simulink model "Micro_Grid_BatteryCharging"  (R2024b)
settings: Solver=VariableStepAuto  StartTime=0.0  StopTime=60*3  RelTol=1e-3
undefined symbols (not defined in the file or in its folder): Acid, Lead
libraries: spsSeriesRLCBranchLib x15, spsVoltageMeasurementLib x9, spsThreePhaseSourceLib x3, spsUniversalBridgeLib x3, spsThreePhaseSeriesRLCBranchLib x2, spsCurrentMeasurementLib x2, spsPWMGenerator2LevelLib x2, spsBreakerLib x2, spsThreePhaseVIMeasurementLib x1, spsBatteryLib x1, slpidlib x1, spsSawtoothGeneratorLib x1
settings Model: SimulationMode=accelerator  Creator=haima  LastModifiedBy=haima

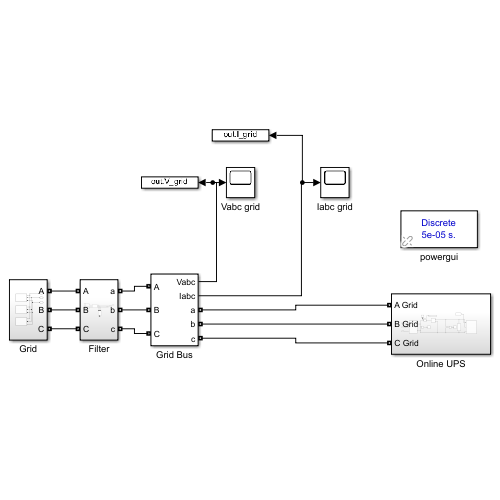
[thumbnail: Simulink's stored preview of the top-level diagram]
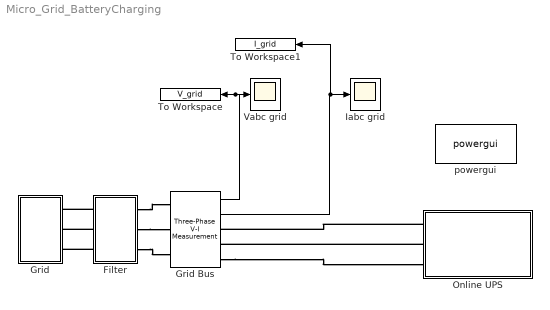
== system Micro_Grid_BatteryCharging ==
  Filter : Subsystem
  Grid : Subsystem
  Grid Bus : spsThreePhaseVIMeasurementLib/Three-Phase V-I Measurement  VoltageMeasurement=phase-to-ground  SetLabelV=off  LabelV=Vabc  Vpu=off  VpuLL=off  CurrentMeasurement=yes  SetLabelI=off  LabelI=Iabc  Ipu=off  Pbase=100e6  Vbase=500e3  OutputType=Complex  PhasorSimulation=off  PSBequivalent=0
  Iabc grid : Scope
  Online UPS : Subsystem
  To Workspace : ToWorkspace  VariableName=V_grid  SaveFormat=Timeseries  SampleTime=-1
  To Workspace1 : ToWorkspace  VariableName=I_grid  SaveFormat=Timeseries  SampleTime=-1
  Vabc grid : Scope
  powergui : spspowerguiLib/powergui  Priority=1  SimulationMode=Discrete  SampleTime=50e-6  frequency=60  Iterations=50  frequencyindice=50  Pbase=100e6  ErrMax=1e-4  UnitsV=kV  UnitsW=MW  buscounter=0  FunctionMessages=off  echomessages=off  EnableUseOfTLC=off  CurrentSourceSwitches=off  DisableSnubberDevices=off  DisableRonSwitches=off  DisableVfSwitches=off  DisplayEquations=off  AutomaticDiscreteSolvers=off  SolverType=Tustin/Backward Euler (TBE)  Interpol=off  ExternalGateDelay=off  methode=off  Ts=100  x0status=blocks  SPID=on  SwTol=0  HookPort=off  NonlinearTolerance=1e-4  nMaxIteration=100  ContinueOnMaxIteration=off  RestoreLinks=warning  ResistiveCurrentMeasurement=off  Frange=[0:2:500]  Ylog=off  Xlog=on  ShowGrid=off  save=off  variable=ZData  structure=0  ZoomFFT=off  StartTime=0.0  cycles=1  DisplayStyle=1  fundamental=60  FreqAxis=off  MaxFrequency=1000  frequencyindicesteady=1  RmsSteady=1  display=off
  wires:
  Grid Bus/2 -> To Workspace1/1, Iabc grid/1
  Grid Bus/1 -> Vabc grid/1, To Workspace/1
  connections:
  Online UPS/LConn1 -- Grid Bus/RConn1
  Grid Bus/RConn3 -- Online UPS/LConn3
  Filter/RConn1 -- Grid Bus/LConn1
  Filter/LConn2 -- Grid/RConn2
  Filter/RConn3 -- Grid Bus/LConn3
  Online UPS/LConn2 -- Grid Bus/RConn2
  Filter/LConn1 -- Grid/RConn1
  Filter/RConn2 -- Grid Bus/LConn2
  Filter/LConn3 -- Grid/RConn3

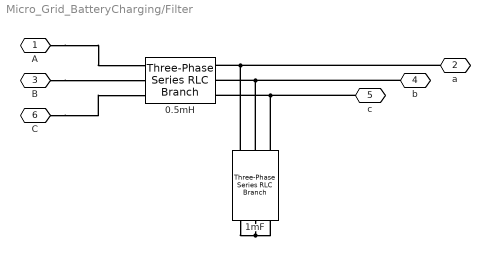
== system Micro_Grid_BatteryCharging/Filter ==
  0.5mH : spsThreePhaseSeriesRLCBranchLib/Three-Phase Series RLC Branch  LConnTagsString=A|B|C  RConnTagsString=A|B|C  BranchType=L  Resistance=1  Inductance=500e-6  Capacitance=1e-6  Measurements=None
  1mF : spsThreePhaseSeriesRLCBranchLib/Three-Phase Series RLC Branch  LConnTagsString=A|B|C  RConnTagsString=A|B|C  BranchType=C  Resistance=1  Inductance=1e-3  Capacitance=100e-6  Measurements=None
  A : PMIOPort  Side=Left
  a : PMIOPort  Port=2  Side=Right
  B : PMIOPort  Port=3  Side=Left
  b : PMIOPort  Port=4  Side=Right
  c : PMIOPort  Port=5  Side=Right
  C : PMIOPort  Port=6  Side=Left
  connections:
  1mF/LConn2 -- 0.5mH/RConn2 -- b/RConn1
  A/RConn1 -- 0.5mH/LConn1
  1mF/RConn1 -- 1mF/RConn3 -- 1mF/RConn2
  1mF/LConn1 -- 0.5mH/RConn1 -- a/RConn1
  C/RConn1 -- 0.5mH/LConn3
  1mF/LConn3 -- 0.5mH/RConn3 -- c/RConn1
  B/RConn1 -- 0.5mH/LConn2

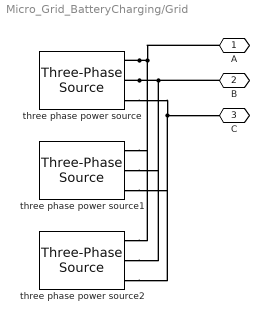
== system Micro_Grid_BatteryCharging/Grid ==
  three phase power source : spsThreePhaseSourceLib/Three-Phase Source  InternalConnection=Yg  VoltagePhases=off  Voltage=380  PhaseAngle=0  Voltage_phases=[25e3 25e3 25e3]/sqrt(3)  PhaseAngles_phases=[0 -120 +120]  Frequency=50  NonIdealSource=on  SpecifyImpedance=off  Resistance=0.8929  Inductance=16.58e-3  ShortCircuitLevel=100e6  BaseVoltage=380  XRratio=7  BusType=PV  Pref=200e6  Qref=0  Prefabc=[10e3, 10e3, 10e3]  Qrefabc=[0, 0, 0]  Qmin=-inf  Qmax=inf
  three phase power source1 : spsThreePhaseSourceLib/Three-Phase Source  InternalConnection=Yg  VoltagePhases=off  Voltage=380  PhaseAngle=0  Voltage_phases=[25e3 25e3 25e3]/sqrt(3)  PhaseAngles_phases=[0 -120 +120]  Frequency=50  NonIdealSource=on  SpecifyImpedance=off  Resistance=0.8929  Inductance=16.58e-3  ShortCircuitLevel=100e6  BaseVoltage=380  XRratio=7  BusType=PV  Pref=200e6  Qref=0  Prefabc=[10e3, 10e3, 10e3]  Qrefabc=[0, 0, 0]  Qmin=-inf  Qmax=inf
  three phase power source2 : spsThreePhaseSourceLib/Three-Phase Source  InternalConnection=Yg  VoltagePhases=off  Voltage=380  PhaseAngle=0  Voltage_phases=[25e3 25e3 25e3]/sqrt(3)  PhaseAngles_phases=[0 -120 +120]  Frequency=50  NonIdealSource=on  SpecifyImpedance=off  Resistance=0.8929  Inductance=16.58e-3  ShortCircuitLevel=100e6  BaseVoltage=380  XRratio=7  BusType=PV  Pref=200e6  Qref=0  Prefabc=[10e3, 10e3, 10e3]  Qrefabc=[0, 0, 0]  Qmin=-inf  Qmax=inf
  A : PMIOPort  Side=Right
  B : PMIOPort  Port=2  Side=Right
  C : PMIOPort  Port=3  Side=Right
  connections:
  three phase power source/RConn3 -- three phase power source2/RConn3 -- three phase power source1/RConn3 -- C/RConn1
  three phase power source/RConn1 -- A/RConn1 -- three phase power source2/RConn1 -- three phase power source1/RConn1
  three phase power source/RConn2 -- B/RConn1 -- three phase power source2/RConn2 -- three phase power source1/RConn2

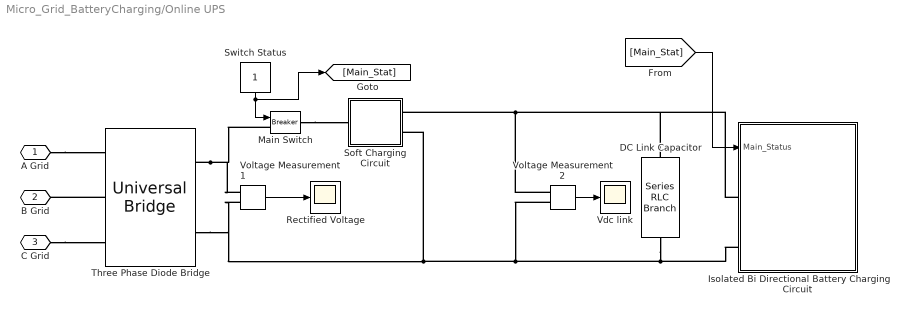
== system Micro_Grid_BatteryCharging/Online UPS ==
  DC Link Capacitor : spsSeriesRLCBranchLib/Series RLC Branch  LConnTagsString=__new0  RConnTagsString=__new0  BranchType=C  Resistance=1  Inductance=1e-3  SetiL0=off  InitialCurrent=0  Capacitance=50e-6  Setx0=off  InitialVoltage=0  Measurements=None
  Isolated Bi Directional Battery Charging Circuit : Subsystem
  Main Switch : spsBreakerLib/Breaker  InitialState=1  SwitchingTimes="[1/60  5/60]"  External=on  BreakerResistance=0.01  SnubberResistance=inf  SnubberCapacitance=inf  Measurements=None  MoreParameters=on  NoBreakLoop=off
  "Rectified Voltage " : Scope
  Soft Charging Circuit : Subsystem
  Switch Status : Constant
  Three Phase Diode Bridge : spsUniversalBridgeLib/Universal Bridge  Arms=3  SnubberResistance=1e5  SnubberCapacitance=inf  Device=Diodes  Ron=1e-3  Lon=0  ForwardVoltages="[  0  0  ]"  ForwardVoltage=0  GTOparameters=[ 10e-6 , 20e-6 ]  IGBTparameters=[ 1e-6 , 2e-6 ]  Measurements=None  Measurements_2=None  converterType=Rectifier
  Vdc link : Scope
  Voltage Measurement1 : spsVoltageMeasurementLib/Voltage Measurement  PhasorSimulation=off  OutputType=Complex  PSBequivalent=0
  Voltage Measurement2 : spsVoltageMeasurementLib/Voltage Measurement  PhasorSimulation=off  OutputType=Complex  PSBequivalent=0
  A Grid : PMIOPort  Side=Left
  B Grid : PMIOPort  Port=2  Side=Left
  C Grid : PMIOPort  Port=3  Side=Left
  wires:
  Voltage Measurement2/1 -> Vdc link/1
  Switch Status/1 -> [Main_Stat], Main Switch/1
  [Main_Stat] -> Isolated Bi Directional Battery Charging Circuit/1(Main_Status)
  Voltage Measurement1/1 -> "Rectified Voltage "/1
  connections:
  DC Link Capacitor/RConn1 -- Isolated Bi Directional Battery Charging Circuit/LConn2 -- Three Phase Diode Bridge/RConn2 -- Voltage Measurement1/LConn2 -- Soft Charging Circuit/RConn2 -- Voltage Measurement2/LConn2
  Voltage Measurement2/LConn1 -- DC Link Capacitor/LConn1 -- Isolated Bi Directional Battery Charging Circuit/LConn1 -- Soft Charging Circuit/RConn1
  C Grid/RConn1 -- Three Phase Diode Bridge/LConn3
  Three Phase Diode Bridge/RConn1 -- Main Switch/LConn1 -- Voltage Measurement1/LConn1
  Main Switch/RConn1 -- Soft Charging Circuit/LConn1
  Three Phase Diode Bridge/LConn2 -- B Grid/RConn1
  A Grid/RConn1 -- Three Phase Diode Bridge/LConn1

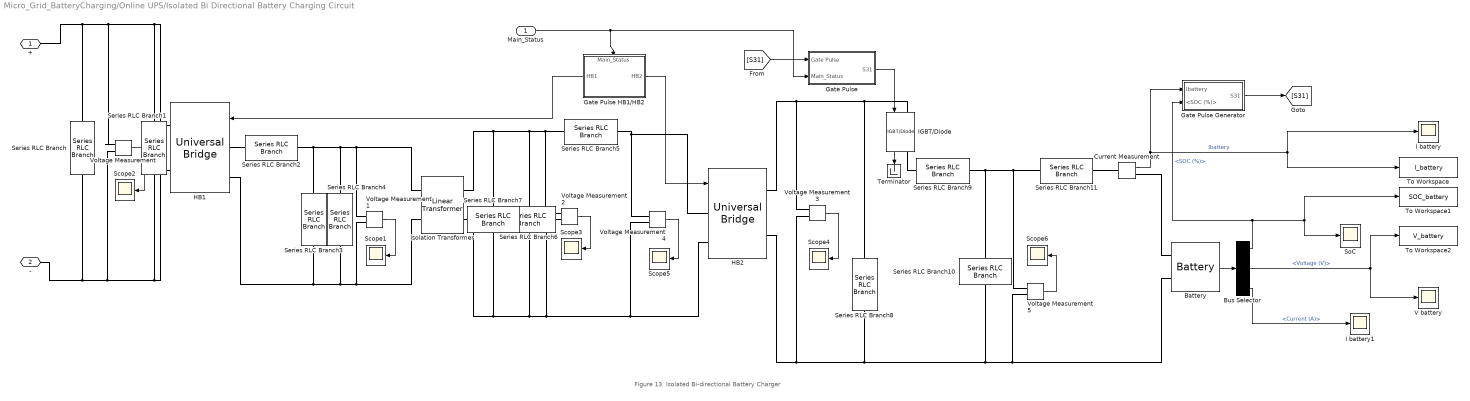
== system Micro_Grid_BatteryCharging/Online UPS/Isolated Bi Directional Battery Charging Circuit ==
  note: Figure 13. Isolated Bi-directional Battery Charger
  Main_Status : Inport
  Battery : spsBatteryLib/Battery  BatType=Lead-Acid  NomV=12  NomQ=14  SOC=30  Batt_Tr=30  PresetModel=on  MaxQ=14.5833  MinV=9  FullV=13.0658  Dis_rate=2.8  R=0.0085714  Normal_OP=4.3439  expZone="[12.2171    0.0466667]"
  Bus Selector : BusSelector  OutputSignals=SOC (%),Voltage (V),Current (A)
  Current Measurement : spsCurrentMeasurementLib/Current Measurement  PhasorSimulation=off  OutputType=Complex  PSBequivalent=0
  Gate Pulse : Subsystem
  Gate Pulse HB1/HB2 : Subsystem
      settings: PortSchema="{\"entries\":[{\"content\":{\"sides\":[{\"content\":{\"connectorIds\":[\"Out2\"]},\"type\":\"ConnectorPlacement.EquallySpacedRectSide\",\"uuid\":\"1234e2fb-321d-4fcf-8e53-b8d56895d88c\"},{\"content\":{\"connectorIds\":[\"Out1\"],\"side\":\"RIGHT\"},\"type\":\"ConnectorPlacement.EquallySpacedRectSide\",\"uuid\":\"c3f79607-e652-4b89-92d0-d6f199718302\"},{\"content\":{\"connectorIds\":[\"In1\"],\"side\":\"TOP\"},\"type\":\"ConnectorPlacement.EquallySpacedRectSide\",\"uuid\":\"8d957198-eefe-4d8f-8635-25a2677fe138\"}]},\"type\":\"ConnectorPlacement.EquallySpacedConnector\",\"uuid\":\"571601be-3060-4c2f-a4a4-d5c9aeeae6bc\"}],\"packageUris\":[\"http://schema.mathworks.com/mf0/Connector/R2020b\"],\"version\":\"1.0\"}"
  Gate Pulse Generator : Subsystem
  HB1 : spsUniversalBridgeLib/Universal Bridge  Arms=2  SnubberResistance=1e5  SnubberCapacitance=inf  Device=IGBT / Diodes  Ron=1e-3  Lon=0  ForwardVoltages="[  0  0.8  ]"  ForwardVoltage=0  GTOparameters=[ 10e-6 , 20e-6 ]  IGBTparameters=[ 1e-6 , 2e-6 ]  Measurements=None  Measurements_2=None  converterType=Rectifier
  HB2 : spsUniversalBridgeLib/Universal Bridge  Arms=2  SnubberResistance=1e5  SnubberCapacitance=inf  Device=IGBT / Diodes  Ron=1e-3  Lon=0  ForwardVoltages="[  0  0.8  ]"  ForwardVoltage=0  GTOparameters=[ 10e-6 , 20e-6 ]  IGBTparameters=[ 1e-6 , 2e-6 ]  Measurements=None  Measurements_2=None  converterType=Rectifier
  I battery : Scope
  I battery1 : Scope
  IGBT/Diode : spsIGBTDiodeLib/IGBT//Diode  Ron=1e-3  Rs=1e5  Cs=inf  Measurements=on
  Isolation Transformer : spsLinearTransformerLib/Linear Transformer  UNITS=pu  NominalPower=[ 250e6 50 ]  winding1=[7.35e+05 0.002 0.08]  winding2=[3.15e+05 0.002 0.08]  ThreeWindings=off  winding3=[3.15e+05 0.002 0.08]  RmLm=[499.98 500]  Measurements=None  DataType=off
  Scope{1..6} (6 alike) : Scope
  Series RLC Branch : spsSeriesRLCBranchLib/Series RLC Branch  LConnTagsString=__new0  RConnTagsString=__new0  BranchType=C  Resistance=1  Inductance=1e-3  SetiL0=off  InitialCurrent=0  Capacitance=1e-2  Setx0=off  InitialVoltage=0  Measurements=None
  Series RLC Branch1 : spsSeriesRLCBranchLib/Series RLC Branch  LConnTagsString=__new0  RConnTagsString=__new0  BranchType=R  Resistance=10000000000  Inductance=1e-3  SetiL0=off  InitialCurrent=0  Capacitance=1e-6  Setx0=off  InitialVoltage=0  Measurements=None
  Series RLC Branch10 : spsSeriesRLCBranchLib/Series RLC Branch  LConnTagsString=__new0  RConnTagsString=__new0  BranchType=C  Resistance=1  Inductance=1e-3  SetiL0=off  InitialCurrent=0  Capacitance=1.56e-3  Setx0=off  InitialVoltage=0  Measurements=None
  Series RLC Branch11 : spsSeriesRLCBranchLib/Series RLC Branch  LConnTagsString=__new0  RConnTagsString=__new0  BranchType=R  Resistance=1  Inductance=1e-3  SetiL0=off  InitialCurrent=0  Capacitance=1e-6  Setx0=off  InitialVoltage=0  Measurements=None
  Series RLC Branch2 : spsSeriesRLCBranchLib/Series RLC Branch  LConnTagsString=__new0  RConnTagsString=__new0  BranchType=L  Resistance=1  Inductance=1e-3  SetiL0=off  InitialCurrent=0  Capacitance=1e-6  Setx0=off  InitialVoltage=0  Measurements=None
  Series RLC Branch3 : spsSeriesRLCBranchLib/Series RLC Branch  LConnTagsString=__new0  RConnTagsString=__new0  BranchType=C  Resistance=1  Inductance=1e-3  SetiL0=off  InitialCurrent=0  Capacitance=1e-5  Setx0=off  InitialVoltage=0  Measurements=None
  Series RLC Branch4 : spsSeriesRLCBranchLib/Series RLC Branch  LConnTagsString=__new0  RConnTagsString=__new0  BranchType=R  Resistance=100  Inductance=1e-3  SetiL0=off  InitialCurrent=0  Capacitance=1e-5  Setx0=off  InitialVoltage=0  Measurements=None
  Series RLC Branch5 : spsSeriesRLCBranchLib/Series RLC Branch  LConnTagsString=__new0  RConnTagsString=__new0  BranchType=L  Resistance=1  Inductance=1e-3  SetiL0=off  InitialCurrent=0  Capacitance=1e-6  Setx0=off  InitialVoltage=0  Measurements=None
  Series RLC Branch6 : spsSeriesRLCBranchLib/Series RLC Branch  LConnTagsString=__new0  RConnTagsString=__new0  BranchType=C  Resistance=1  Inductance=1e-3  SetiL0=off  InitialCurrent=0  Capacitance=1e-5  Setx0=off  InitialVoltage=0  Measurements=None
  Series RLC Branch7 : spsSeriesRLCBranchLib/Series RLC Branch  LConnTagsString=__new0  RConnTagsString=__new0  BranchType=R  Resistance=100  Inductance=1e-3  SetiL0=off  InitialCurrent=0  Capacitance=1e-5  Setx0=off  InitialVoltage=0  Measurements=None
  Series RLC Branch8 : spsSeriesRLCBranchLib/Series RLC Branch  LConnTagsString=__new0  RConnTagsString=__new0  BranchType=C  Resistance=1  Inductance=1e-3  SetiL0=off  InitialCurrent=0  Capacitance=5e-3  Setx0=off  InitialVoltage=0  Measurements=None
  Series RLC Branch9 : spsSeriesRLCBranchLib/Series RLC Branch  LConnTagsString=__new0  RConnTagsString=__new0  BranchType=L  Resistance=1  Inductance=500e-3  SetiL0=off  InitialCurrent=0  Capacitance=1e-6  Setx0=off  InitialVoltage=0  Measurements=None
  SoC : Scope
  Terminator : Terminator
  To Workspace : ToWorkspace  VariableName=I_battery  SaveFormat=Timeseries  SampleTime=-1
  To Workspace1 : ToWorkspace  VariableName=SOC_battery  SaveFormat=Timeseries  SampleTime=-1
  To Workspace2 : ToWorkspace  VariableName=V_battery  SaveFormat=Timeseries  SampleTime=-1
  V battery : Scope
  Voltage Measurement{,1..5} (6 alike) : spsVoltageMeasurementLib/Voltage Measurement  PhasorSimulation=off  OutputType=Complex  PSBequivalent=0
  + : PMIOPort  Side=Left
  - : PMIOPort  Port=2  Side=Left
  wires:
  Voltage Measurement5/1 -> Scope6/1
  Gate Pulse Generator/1(S31) -> [S31]
  Bus Selector/1 -> To Workspace1/1, SoC/1, Gate Pulse Generator/2(<SOC (%)>)  "<SOC (%)>"
  Voltage Measurement4/1 -> Scope5/1
  Battery/1 -> Bus Selector/1
  Voltage Measurement3/1 -> Scope4/1
  Gate Pulse HB1/HB2/1(HB2) -> HB2/1
  Bus Selector/2 -> To Workspace2/1, V battery/1  "<Voltage (V)>"
  Voltage Measurement2/1 -> Scope3/1
  Voltage Measurement/1 -> Scope2/1
  Voltage Measurement1/1 -> Scope1/1
  IGBT/Diode/1 -> Terminator/1
  Gate Pulse HB1/HB2/2(HB1) -> HB1/1
  Current Measurement/1 -> Gate Pulse Generator/1(Ibattery), I battery/1, To Workspace/1  "Ibattery"
  Bus Selector/3 -> I battery1/1  "<Current (A)>"
  Main_Status/1 -> Gate Pulse HB1/HB2/1(Main_Status), Gate Pulse/2(Main_Status)
  [S31] -> Gate Pulse/1(Gate Pulse)
  Gate Pulse/1(S31) -> IGBT/Diode/1
  connections:
  Battery/LConn1 -- Current Measurement/RConn1
  Series RLC Branch10/RConn1 -- Battery/LConn2 -- Voltage Measurement5/LConn2 -- Voltage Measurement3/LConn2 -- HB2/RConn2 -- Series RLC Branch8/RConn1
  -/RConn1 -- Series RLC Branch/RConn1 -- Series RLC Branch1/RConn1 -- HB1/RConn2 -- Voltage Measurement/LConn2
  Series RLC Branch10/LConn1 -- Series RLC Branch11/RConn1 -- Voltage Measurement5/LConn1 -- Series RLC Branch9/LConn1
  Current Measurement/LConn1 -- Series RLC Branch11/LConn1
  HB2/LConn2 -- Voltage Measurement4/LConn2 -- Voltage Measurement2/LConn2 -- Series RLC Branch6/RConn1 -- Series RLC Branch7/RConn1 -- Isolation Transformer/RConn2
  Series RLC Branch9/RConn1 -- IGBT/Diode/RConn1
  HB1/RConn1 -- Series RLC Branch1/LConn1 -- Series RLC Branch/LConn1 -- +/RConn1 -- Voltage Measurement/LConn1
  Voltage Measurement1/LConn1 -- Series RLC Branch3/LConn1 -- Series RLC Branch2/RConn1 -- Series RLC Branch4/LConn1 -- Isolation Transformer/LConn1
  Series RLC Branch4/RConn1 -- Voltage Measurement1/LConn2 -- Isolation Transformer/LConn2 -- Series RLC Branch3/RConn1 -- HB1/LConn2
  HB1/LConn1 -- Series RLC Branch2/LConn1
  HB2/LConn1 -- Series RLC Branch5/LConn1 -- Voltage Measurement4/LConn1
  IGBT/Diode/LConn1 -- Series RLC Branch8/LConn1 -- Voltage Measurement3/LConn1 -- HB2/RConn1
  Series RLC Branch7/LConn1 -- Series RLC Branch5/RConn1 -- Voltage Measurement2/LConn1 -- Series RLC Branch6/LConn1 -- Isolation Transformer/RConn1

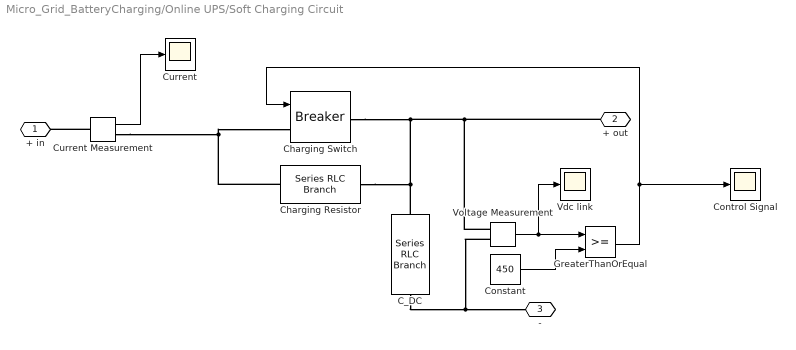
== system Micro_Grid_BatteryCharging/Online UPS/Soft Charging Circuit ==
  C_DC : spsSeriesRLCBranchLib/Series RLC Branch  LConnTagsString=__new0  RConnTagsString=__new0  BranchType=C  Resistance=1  Inductance=1e-3  SetiL0=off  InitialCurrent=0  Capacitance=6.4e-3  Setx0=off  InitialVoltage=0  Measurements=None
  Charging Resistor : spsSeriesRLCBranchLib/Series RLC Branch  LConnTagsString=__new0  RConnTagsString=__new0  BranchType=R  Resistance=10  Inductance=16.8e-3  SetiL0=off  InitialCurrent=0  Capacitance=1e-6  Setx0=off  InitialVoltage=0  Measurements=None
  Charging Switch : spsBreakerLib/Breaker  InitialState=0  SwitchingTimes="[1/60  5/60]"  External=on  BreakerResistance=0.01  SnubberResistance=inf  SnubberCapacitance=inf  Measurements=None  MoreParameters=on  NoBreakLoop=off
  Constant : Constant  Value=450
  Control Signal : Scope
  Current : Scope
  Current Measurement : spsCurrentMeasurementLib/Current Measurement  PhasorSimulation=off  OutputType=Complex  PSBequivalent=0
  GreaterThanOrEqual : RelationalOperator  OutDataTypeStr=boolean  RndMeth=Simplest  InputSameDT=off
  Vdc link : Scope
  Voltage Measurement : spsVoltageMeasurementLib/Voltage Measurement  PhasorSimulation=off  OutputType=Complex  PSBequivalent=0
  + in : PMIOPort  Side=Left
  + out : PMIOPort  Port=2  Side=Right
  - : PMIOPort  Port=3  Side=Right
  wires:
  Voltage Measurement/1 -> Vdc link/1, GreaterThanOrEqual/1
  Constant/1 -> GreaterThanOrEqual/2
  GreaterThanOrEqual/1 -> Control Signal/1, Charging Switch/1
  Current Measurement/1 -> Current/1
  connections:
  Charging Resistor/LConn1 -- Current Measurement/RConn1 -- Charging Switch/LConn1
  Charging Switch/RConn1 -- + out/RConn1 -- Voltage Measurement/LConn1 -- C_DC/LConn1 -- Charging Resistor/RConn1
  C_DC/RConn1 -- Voltage Measurement/LConn2 -- -/RConn1
  Current Measurement/LConn1 -- + in/RConn1

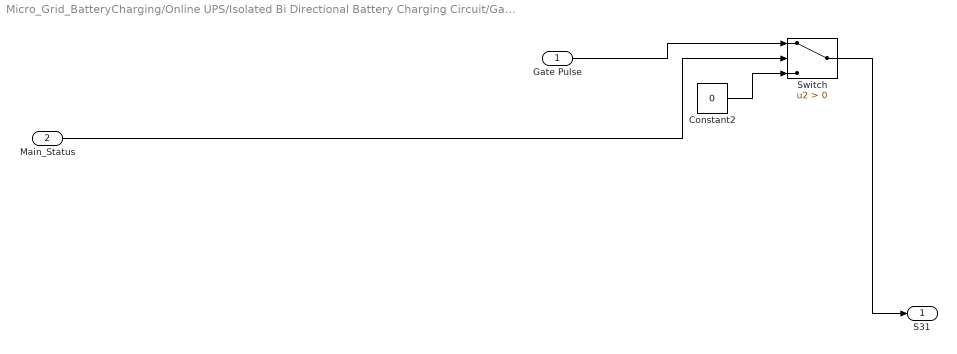
== system Micro_Grid_BatteryCharging/Online UPS/Isolated Bi Directional Battery Charging Circuit/Gate Pulse ==
  Gate Pulse : Inport
  Main_Status : Inport  Port=2
  Constant2 : Constant  Value=0
  Switch : Switch  Criteria=u2 > Threshold  SaturateOnIntegerOverflow=off  InputSameDT=off
  S31 : Outport
  wires:
  Switch/1 -> S31/1
  Gate Pulse/1 -> Switch/1
  Main_Status/1 -> Switch/2
  Constant2/1 -> Switch/3

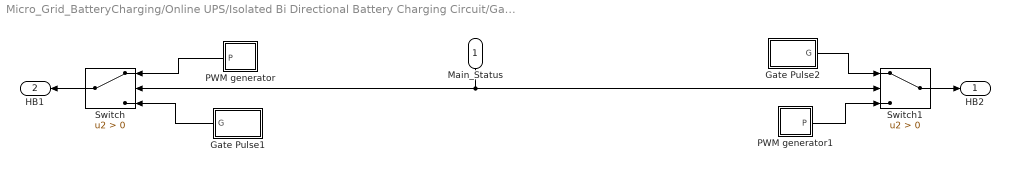
== system Micro_Grid_BatteryCharging/Online UPS/Isolated Bi Directional Battery Charging Circuit/Gate Pulse HB1//HB2 ==
  Main_Status : Inport
  Gate Pulse1 : Subsystem
  Gate Pulse2 : Subsystem
  PWM generator : Subsystem
      settings: PortSchema="{\"entries\":[{\"content\":{\"sides\":[{\"content\":{\"connectorIds\":[\"Out1\"]},\"type\":\"ConnectorPlacement.EquallySpacedRectSide\",\"uuid\":\"807d608c-be67-4f89-a244-8e5044f7f1fa\"},{\"content\":{\"side\":\"RIGHT\"},\"type\":\"ConnectorPlacement.EquallySpacedRectSide\",\"uuid\":\"ae9c9264-81d1-4b5c-861e-635da60d63e0\"},{\"content\":{\"side\":\"TOP\"},\"type\":\"ConnectorPlacement.EquallySpacedRectSide\",\"uuid\":\"146f21cb-b82e-455a-b0a2-4badca4c67c8\"}]},\"type\":\"ConnectorPlacement.EquallySpacedConnector\",\"uuid\":\"ec685afc-0591-41aa-a445-2815616301aa\"}],\"packageUris\":[\"http://schema.mathworks.com/mf0/Connector/R2020b\"],\"version\":\"1.0\"}"
  PWM generator1 : Subsystem
      settings: PortSchema="{\"entries\":[{\"content\":{\"sides\":[{\"content\":{\"connectorIds\":[\"Out1\"]},\"type\":\"ConnectorPlacement.EquallySpacedRectSide\",\"uuid\":\"807d608c-be67-4f89-a244-8e5044f7f1fa\"},{\"content\":{\"side\":\"RIGHT\"},\"type\":\"ConnectorPlacement.EquallySpacedRectSide\",\"uuid\":\"ae9c9264-81d1-4b5c-861e-635da60d63e0\"},{\"content\":{\"side\":\"TOP\"},\"type\":\"ConnectorPlacement.EquallySpacedRectSide\",\"uuid\":\"146f21cb-b82e-455a-b0a2-4badca4c67c8\"}]},\"type\":\"ConnectorPlacement.EquallySpacedConnector\",\"uuid\":\"ec685afc-0591-41aa-a445-2815616301aa\"}],\"packageUris\":[\"http://schema.mathworks.com/mf0/Connector/R2020b\"],\"version\":\"1.0\"}"
  Switch : Switch  Criteria=u2 > Threshold  SaturateOnIntegerOverflow=off  InputSameDT=off
  Switch1 : Switch  Criteria=u2 > Threshold  SaturateOnIntegerOverflow=off  InputSameDT=off
  HB2 : Outport
  HB1 : Outport  Port=2
  wires:
  Gate Pulse1/1(G) -> Switch/3
  Main_Status/1 -> Switch1/2, Switch/2
  Switch1/1 -> HB2/1
  PWM generator/1(P) -> Switch/1
  Switch/1 -> HB1/1
  PWM generator1/1(P) -> Switch1/3
  Gate Pulse2/1(G) -> Switch1/1

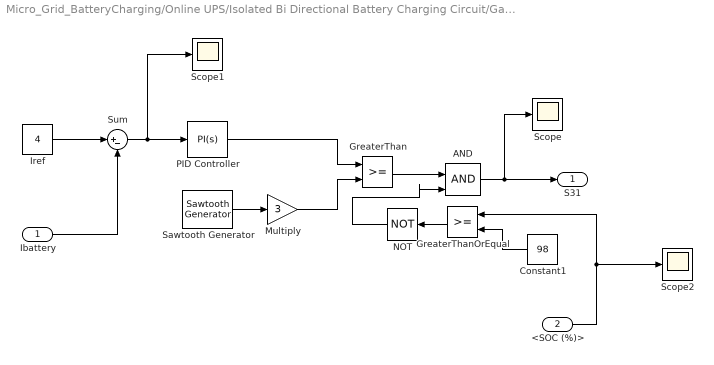
== system Micro_Grid_BatteryCharging/Online UPS/Isolated Bi Directional Battery Charging Circuit/Gate Pulse Generator ==
  Ibattery : Inport
  <SOC (%)> : Inport  Port=2
  AND : Logic  IconShape=distinctive  AllPortsSameDT=off  OutDataTypeStr=boolean
  Constant1 : Constant  Value=98
  GreaterThan : RelationalOperator  OutDataTypeStr=boolean  RndMeth=Simplest  InputSameDT=off
  GreaterThanOrEqual : RelationalOperator  OutDataTypeStr=boolean  RndMeth=Simplest  InputSameDT=off
  Iref : Constant  Value=4
  Multiply : Gain  Gain=3
  NOT : Logic  Operator=NOT  IconShape=distinctive  AllPortsSameDT=off  OutDataTypeStr=boolean
  PID Controller : slpidlib/PID Controller  Controller=PI  Form=Parallel  TimeDomain=Continuous-time  UseExternalTs=off  SampleTime=-1  IntegratorMethod=Forward Euler  FilterMethod=Forward Euler  ControllerParametersSource=internal  P=1  I=1  UseKiTs=off  D=0  UseExternalDerivativeSource=off  N=100  UseFilter=on  TunerSelectOption=Transfer Function Based (PID Tuner App)  InitialConditionSource=internal  InitialConditionForIntegrator=0  InitialConditionForFilter=0  DifferentiatorICPrevScaledInput=0  ExternalReset=none  TrackingMode=off  Kt=1  LimitOutput=off  SatLimitsSource=internal  UpperSaturationLimit=inf  LowerSaturationLimit=-inf  LinearizeAsGain=on  AntiWindupMode=none  Kb=1  LimitIntegrator=off  UpperIntegratorSaturationLimit=inf  LowerIntegratorSaturationLimit=-inf  POutMin=[]  POutMax=[]  IOutMin=[]  IOutMax=[]  DOutMin=[]  DOutMax=[]  NOutMin=[]  NOutMax=[]  SumOutMin=[]  SumOutMax=[]  SaturationOutMin=[]  SaturationOutMax=[]  PParamMin=[]  PParamMax=[]  IParamMin=[]  IParamMax=[]  DParamMin=[]  DParamMax=[]  NParamMin=[]  NParamMax=[]  KbParamMin=[]  KbParamMax=[]  KtParamMin=[]  KtParamMax=[]  KbOutMin=[]  KbOutMax=[]  KtOutMin=[]  KtOutMax=[]  IntegratorOutMin=[]  IntegratorOutMax=[]  FilterOutMin=[]  FilterOutMax=[]  SumI1OutMin=[]  SumI1OutMax=[]  SumI2OutMin=[]  SumI2OutMax=[]  SumI3OutMin=[]  SumI3OutMax=[]  SumI4OutMin=[]  SumI4OutMax=[]  SumDOutMin=[]  SumDOutMax=[]  DifferentiatorOutMin=[]  DifferentiatorOutMax=[]  FilterDiffOutCoefMin=[]  FilterDiffOutCoefMax=[]  ReciprocalOutMin=[]  ReciprocalOutMax=[]  SumDenOutMin=[]  SumDenOutMax=[]  SumNumOutMin=[]  SumNumOutMax=[]  DivideOutMin=[]  DivideOutMax=[]  UdiffTsProdOutMin=[]  UdiffTsProdOutMax=[]  NTsProdOutMin=[]  NTsProdOutMax=[]  UintegralTsProdOutMin=[]  UintegralTsProdOutMax=[]  UngainTsProdOutMin=[]  UngainTsProdOutMax=[]  ClampingZeroOutDataTypeStr=Inherit: Inherit via back propagation  ClampingZeroOutMin=[]  ClampingZeroOutMax=[]  FilterDenConstantOutDataTypeStr=Inherit: Inherit via back propagation  FilterDenConstantOutMin=[]  FilterDenConstantOutMax=[]  PCopyOutDataTypeStr=Inherit: Inherit via back propagation  PCopyOutMin=[]  PCopyOutMax=[]  NCopyOutDataTypeStr=Inherit: Inherit via back propagation  NCopyOutMin=[]  NCopyOutMax=[]  IntegratorContinuousStateAttributes=''  IntegratorStateMustResolveToSignalObject=off  IntegratorRTWStateStorageClass=Auto  FilterContinuousStateAttributes=''  FilterStateMustResolveToSignalObject=off  FilterRTWStateStorageClass=Auto  ParallelPVariant=InternalParameters  IdealPVariant=Disabled  IVariant=InternalParameters  DVariant=Disabled  IntegratorVariant=Continuous  SatVariant=Disabled  AWVariant=Passthrough  PCopyVariant=Disabled  TRVariant=Disabled  FdbkBlocksVariant=Forward  IdealPFdbkVariant=Disabled  SatFdbkVariant=Disabled  DerivativeFilterVariant=Disabled  NVariant=Disabled  NCopyVariant=Disabled_SignalSpec  FilterICVariant=Disabled  IntegratorICVariant=InternalICs  ExternalResetVariant=Disabled  TRSumVariant=Passthrough  SumFdbkVariant=Disabled  SumVariant=Sum_PI  TsampFilterVariant=InternalTs  TsampNgainVariant=Passthrough  TsampIntegralVariant=Disabled_SignalSpec  ExternalSaturationOutDataTypeStr=Inherit: Same as second input  DerivativeSourceVariant=Disabled  PreIntVariant=InternalPreInt
  Sawtooth Generator : spsSawtoothGeneratorLib/Sawtooth Generator  Freq=20000  Phase=0  Ts=0
  Scope : Scope
  Scope1 : Scope
  Scope2 : Scope
  Sum : Sum  Inputs=|+-
  S31 : Outport
  wires:
  GreaterThanOrEqual/1 -> NOT/1
  Ibattery/1 -> Sum/2
  Sum/1 -> Scope1/1, PID Controller/1
  Constant1/1 -> GreaterThanOrEqual/2
  PID Controller/1 -> GreaterThan/1
  Iref/1 -> Sum/1
  GreaterThan/1 -> AND/1
  <SOC (%)>/1 -> Scope2/1, GreaterThanOrEqual/1
  NOT/1 -> AND/2
  Sawtooth Generator/1 -> Multiply/1
  AND/1 -> Scope/1, S31/1
  Multiply/1 -> GreaterThan/2

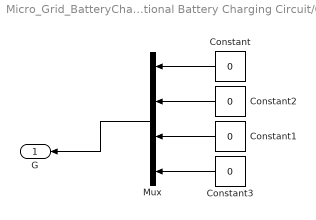
== system Micro_Grid_BatteryCharging/Online UPS/Isolated Bi Directional Battery Charging Circuit/Gate Pulse HB1//HB2/Gate Pulse1 ==
  Constant{,1..3} (4 alike) : Constant  Value=0
  Mux : Mux
  G : Outport
  wires:
  Mux/1 -> G/1
  Constant3/1 -> Mux/4
  Constant1/1 -> Mux/3
  Constant/1 -> Mux/1
  Constant2/1 -> Mux/2

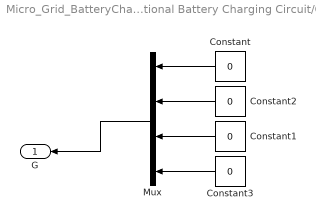
== system Micro_Grid_BatteryCharging/Online UPS/Isolated Bi Directional Battery Charging Circuit/Gate Pulse HB1//HB2/Gate Pulse2 ==
  Constant{,1..3} (4 alike) : Constant  Value=0
  Mux : Mux
  G : Outport
  wires:
  Mux/1 -> G/1
  Constant3/1 -> Mux/4
  Constant1/1 -> Mux/3
  Constant/1 -> Mux/1
  Constant2/1 -> Mux/2

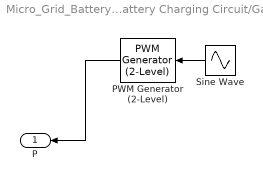
== system Micro_Grid_BatteryCharging/Online UPS/Isolated Bi Directional Battery Charging Circuit/Gate Pulse HB1//HB2/PWM generator ==
  PWM Generator (2-Level) : spsPWMGenerator2LevelLib/PWM Generator (2-Level)  ModulatorType=Single-phase full-bridge (4 pulses)  ModulatorMode=Unsynchronized  Fc=50*100  Pc=0  nF=27  MinMax="[ -1  1 ]"  SamplingTechnique=Natural  ModulatingSignals=off  m=0.8  Freq=60  Phase=0  Ts=0  ShowCarrierOutport=off
  Sine Wave : Sin  Frequency=2*pi*50  SampleTime=0
  P : Outport
  wires:
  PWM Generator (2-Level)/1 -> P/1
  Sine Wave/1 -> PWM Generator (2-Level)/1

== system Micro_Grid_BatteryCharging/Online UPS/Isolated Bi Directional Battery Charging Circuit/Gate Pulse HB1//HB2/PWM generator1 ==
  PWM Generator (2-Level) : spsPWMGenerator2LevelLib/PWM Generator (2-Level)  ModulatorType=Single-phase full-bridge (4 pulses)  ModulatorMode=Unsynchronized  Fc=50*100  Pc=0  nF=27  MinMax="[ -1  1 ]"  SamplingTechnique=Natural  ModulatingSignals=off  m=0.8  Freq=60  Phase=0  Ts=0  ShowCarrierOutport=off
  Sine Wave : Sin  Frequency=2*pi*50  SampleTime=0
  P : Outport
  wires:
  PWM Generator (2-Level)/1 -> P/1
  Sine Wave/1 -> PWM Generator (2-Level)/1
